simulink model "VFM_voltagesag"  (R2025a)
settings: Solver=FixedStepAuto  StartTime=0.0  StopTime=t_end+t_sim_start  FixedStep=Ts  RelTol=1e-3
InitFcn:
  | run VFMPara.m
values from neighbouring files (symbols this model uses):
  Cf = 0.0083    [GFMPara.m]    (also in GFMPara_exp.m = 0.0249; VFMPara.m = 0.02; VFMPara_exp.m = 0.03)
  dt_sag = t_c    [GFMPara.m]    (also in GFMPara_exp.m; PLLpara.m; VFMPara.m; VFMPara_exp.m)
  Lc = 1e-9    (= 1e-09)    [GFMPara.m]    (also in GFMPara_exp.m; PLLpara.m; VFMPara.m; VFMPara_exp.m)
  Lf = 0.0592    [GFMPara.m]    (also in GFMPara_exp.m; PLLpara.m = 0.05; VFMPara.m = 0.05; VFMPara_exp.m = 0.05)
  Lg11 = Xg    [PLLpara.m]    (also in VFMPara.m; VFMPara_exp.m)
  m_gfm = 1/D    [GFMPara.m]    (also in GFMPara_exp.m)
  Rg11 = Rg    [PLLpara.m]    (also in VFMPara.m; VFMPara_exp.m)
  Sbase = 1    [GFMPara.m]    (also in GFMPara_exp.m; PLLpara.m; VFMPara.m; VFMPara_exp.m)
  Scale_ki_v = 20    [GFMPara.m]    (also in GFMPara_exp.m; VFMPara.m; VFMPara_exp.m)
  t0_sag = t_sim_start +t_start    [GFMPara.m]    (also in GFMPara_exp.m; PLLpara.m = 20; VFMPara.m; VFMPara_exp.m = 20)
  Ts = 1/Fs    (= 1e-05)    [GFMPara.m]    (also in GFMPara_exp.m = 1e-06; PLLpara.m = 1e-06; VFMPara.m = 5e-06; VFMPara_exp.m = 1e-06)
  v_sag = Ug_fault    [GFMPara.m]    (also in GFMPara_exp.m; PLLpara.m; VFMPara.m; VFMPara_exp.m)
  Vbase = 1    [GFMPara.m]    (also in GFMPara_exp.m; PLLpara.m; VFMPara.m; VFMPara_exp.m)
  Vdc_ref = 2.5    [GFMPara_exp.m]
  w_droop = D/J    [GFMPara.m]    (also in GFMPara_exp.m; VFMPara.m = 314.159265359; VFMPara_exp.m = 314.159265359)
  w_i_GFM = 2000*2*pi    (= 12566.3706144)    [GFMPara.m]    (also in GFMPara_exp.m = 9424.77796077; VFMPara.m = 9424.77796077; VFMPara_exp.m = 9424.77796077)
  w_v_GFM = 800 *2*pi    (= 5026.54824574)    [GFMPara.m]    (also in GFMPara_exp.m = 3141.59265359; VFMPara.m = 3141.59265359; VFMPara_exp.m = 3141.59265359)
  Wbase = 2*pi*50    (= 314.159265359)    [GFMPara.m]    (also in GFMPara_exp.m; PLLpara.m; VFMPara.m; VFMPara_exp.m)
  Zbase = Vbase/Ibase    (= 1)    [GFMPara.m]    (also in GFMPara_exp.m; PLLpara.m; VFMPara.m; VFMPara_exp.m)
undefined symbols (not defined in the file or in its folder): DiscIntNeverNeededParam, dspblkCoreblockFVToolHelper, gcbh, initial, Kip, Kpp, Pin, Y_dc
libraries: spsVoltageMeasurementLib x32, spsCurrentMeasurementLib x30, spsControlledVoltageSourceLib x12, spsThreePhaseSeriesRLCBranchLib x9, spsSeriesRLCBranchLib x8, spsControlledCurrentSourceLib x4, spsDCVoltageSourceLib x2, spsDiodeLib x2, spspowerguiLib x1
(part 1 of 2)
settings Model: Creator=admin_user  LastModifiedBy=yifan
settings SolverCC: AlgebraicLoopSolver=TrustRegion
settings DataIOCC: ReturnWorkspaceOutputs=off
settings ModelReferenceCC: EnableRefExpFcnMdlSchedulingChecks=on
settings RTWCC: GPUComputeCapability=3.5  DLArmComputeVersion=19.05

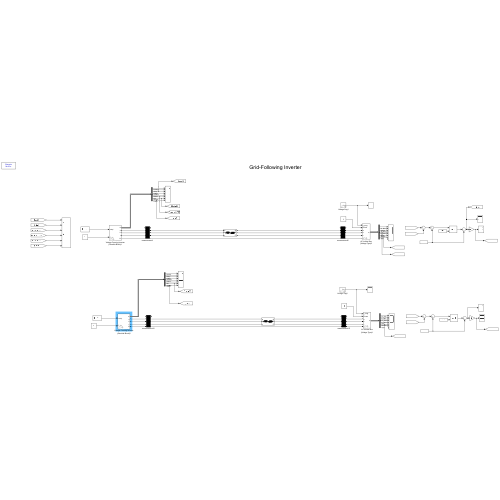
[thumbnail: Simulink's stored preview of the top-level diagram]
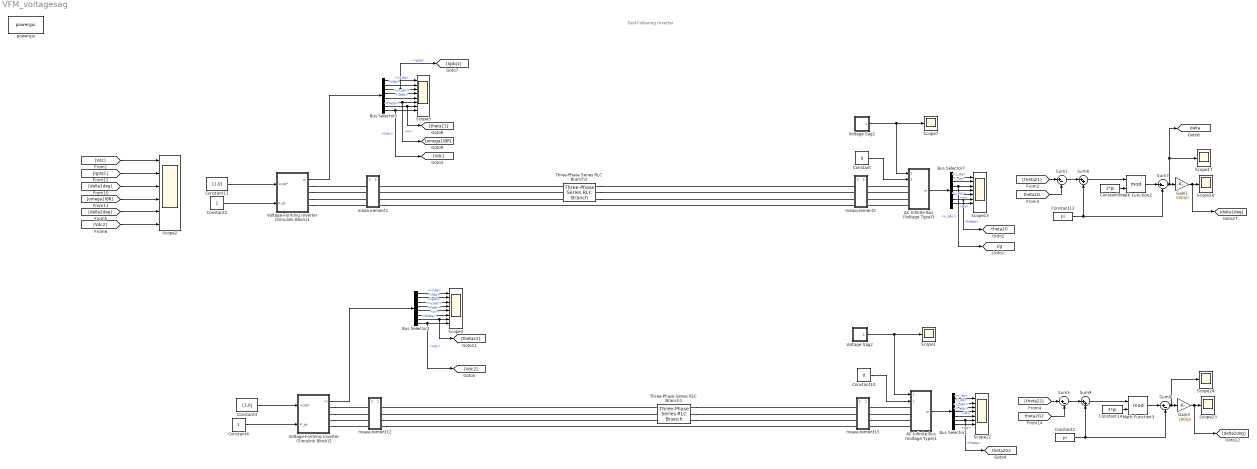
== system VFM_voltagesag ==
  note: Grid-Following Inverter
  AC Infinite Bus (Voltage Type)1 : Subsystem  AncestorBlock=|  mask{Ts=Ts, Sbase=Sbase, Vbase=Vbase, Wbase=Wbase, theta0=0, w=Wbase, R=1e-30}
      | SimplusGT/AC Infinite Bus
      | (Voltage Type)
      mask prompts: Ts "Ts (s), samping period"; Sbase "Sbase (VA), power base"; Vbase "Vbase (V), voltage base"; Wbase "Wbase (rad/s), frequency base"; theta0 "theta0 (rad), initial angle"; w "w (rad/s), frequency"; R "R (Ohm), resistance"
  AC Infinite Bus (Voltage Type)3 : Subsystem  AncestorBlock=|  mask{Ts=Ts, Sbase=Sbase, Vbase=Vbase, Wbase=Wbase, theta0=0, w=Wbase, R=1e-30}
      | SimplusGT/AC Infinite Bus
      | (Voltage Type)
      mask prompts: Ts "Ts (s), samping period"; Sbase "Sbase (VA), power base"; Vbase "Vbase (V), voltage base"; Wbase "Wbase (rad/s), frequency base"; theta0 "theta0 (rad), initial angle"; w "w (rad/s), frequency"; R "R (Ohm), resistance"
  Bus Selector1 : BusSelector  OutputSignals=v_dq,i_dq,v_abc,i_abc,w,theta,pq
  Bus Selector2 : BusSelector  OutputSignals=vcdq,ildq,igdq,vcabc,ilabc,w,theta,Vdc
  Bus Selector5 : BusSelector  OutputSignals=vcdq,ildq,igdq,vcabc,ilabc,w,theta,Vdc
  Bus Selector7 : BusSelector  OutputSignals=v_dq,i_dq,v_abc,i_abc,w,theta,pq
  Constant : Constant  Value=0
  Constant1 : Constant  Value=pi
  Constant10 : Constant  Value=0
  Constant11 : Constant  Value=[1,0]
  Constant12 : Constant  Value=pi
  Constant14 : Constant  Value=2*pi
  Constant2 : Constant
  Constant3 : Constant  Value=[1,0]
  Constant4 : Constant
  Constant9 : Constant  Value=2*pi
  Gain1 : Gain  Gain=180/pi
  Gain3 : Gain  Gain=180/pi
  Math Function2 : Math  Operator=mod  SignedPower=on
  Math Function3 : Math  Operator=mod  SignedPower=on
  Scope{1,7,16..17,23..24} (6 alike) : Scope
      Scope1 settings: ActiveDisplayYMinimum=0.9  ActiveDisplayYMaximum=1.1  DataLoggingVariableName=ScopeData15
      Scope16 settings: ActiveDisplayYMinimum=-0.045003  ActiveDisplayYMaximum=-0.044992  DataLoggingDecimation=10  DataLoggingVariableName=ScopeData6
      Scope17 settings: ActiveDisplayYMinimum=-0.00078544  ActiveDisplayYMaximum=-0.00078526  DataLoggingDecimation=10  DataLoggingVariableName=log_Delta
      Scope23 settings: ActiveDisplayYMinimum=-224.72735  ActiveDisplayYMaximum=224.86411  DataLoggingDecimation=10  DataLoggingVariableName=ScopeData7
      Scope24 settings: ActiveDisplayYMinimum=-3.92678  ActiveDisplayYMaximum=3.92693  DataLoggingDecimation=10  DataLoggingVariableName=log_Delta2
      Scope7 settings: ActiveDisplayYMinimum=0.9  ActiveDisplayYMaximum=1.1
  Scope{3,5,15,22} (4 alike) : Scope  NumInputPorts=8
      Scope15 settings: ActiveDisplayYMinimum=-0.125  ActiveDisplayYMaximum=1.125  DataLoggingVariableName=ScopeData5
      Scope22 settings: ActiveDisplayYMinimum=-0.12499999999999997  ActiveDisplayYMaximum=1.125  DataLoggingVariableName=ScopeData20
      Scope3 settings: ActiveDisplayYMinimum=-0.32470948731946192  ActiveDisplayYMaximum=1.552053078523207  DataLoggingDecimation=10  DataLoggingVariableName=ScopeData3
      Scope5 settings: ActiveDisplayYMinimum=-0.12696977606598872  ActiveDisplayYMaximum=1.1252178168649181  DataLoggingDecimation=10  DataLoggingVariableName=ScopeData2
  Scope2 : Scope  NumInputPorts=6
      settings: TimeSpan=1.5  ActiveDisplayYMinimum=1.8779617654019547  ActiveDisplayYMaximum=3.0300434734077735  DataLoggingDecimation=10
  Sum{1,5,7,9} (4 alike) : Sum  Inputs=|+-
  Sum6 : Sum  Inputs=|++
  Sum8 : Sum  Inputs=|++
  Three-Phase Series RLC Branch1 : spsThreePhaseSeriesRLCBranchLib/Three-Phase Series RLC Branch  LConnTagsString=A|B|C  RConnTagsString=A|B|C  BranchType=RL  Resistance=Rg11*Zbase  Inductance=Lg11*Zbase/Wbase  Capacitance=1/Wbase  Measurements=None
  Three-Phase Series RLC Branch2 : spsThreePhaseSeriesRLCBranchLib/Three-Phase Series RLC Branch  LConnTagsString=A|B|C  RConnTagsString=A|B|C  BranchType=RL  Resistance=Rg11*Zbase  Inductance=Lg11*Zbase/Wbase  Capacitance=1/Wbase  Measurements=None
  Voltage Sag1 : Subsystem  AncestorBlock=SimplusGT/Single Pulse  mask{t0=t0_sag, dt=dt_sag, Am=v_sag}
      mask prompts: t0 "t0 (s), starting time"; dt "dt (s), pulse width"; Am "Am, pulse amplitude"
  Voltage Sag2 : Subsystem  AncestorBlock=SimplusGT/Single Pulse  mask{t0=t0_sag, dt=dt_sag, Am=v_sag}
      mask prompts: t0 "t0 (s), starting time"; dt "dt (s), pulse width"; Am "Am, pulse amplitude"
  Voltage-Forming Inverter (Simulink Block)1 : Subsystem  AncestorBlock=|  mask{Ts=Ts, Sbase=Sbase, Vbase=Vbase, Wbase=Wbase, w_i=w_i_GFM, w_v=w_v_GFM, w_droop=w_droop*1, m=m_gfm, Lf=Lf, Cf=Cf, Lc=Lc, Scale_ki_v=Scale_ki_v}
      | SimplexPS/Grid-Forming Inverter
      | (Simulink Block)
      mask prompts: Ts "Ts (s), sampling period"; Sbase "Sbase (VA), base power"; Vbase "Vbase (V), base voltage"; Wbase "Wbase (rad/s), base frequency"; w_i "w_i (rad/s), current-loop bandwidth"; w_v "w_v (rad/s), voltage-loop bandwidth"; w_droop "w_droop (rad/s), droop bandwidth"; m "m (pu), frequency droop gain"; Lf "Lf (pu), LCL filter"; Cf "Cf (pu), LCL filter"; Lc "Lc (pu), LCL filter"
  Voltage-Forming Inverter (Simulink Block)2 : Subsystem  AncestorBlock=|  mask{Ts=Ts, Sbase=Sbase, Vbase=Vbase, Wbase=Wbase, w_i=w_i_GFM, w_v=w_v_GFM, w_droop=w_droop*1, m=m_gfm, Lf=Lf, Cf=Cf, Lc=Lc, Scale_ki_v=Scale_ki_v}
      | SimplexPS/Grid-Forming Inverter
      | (Simulink Block)
      mask prompts: Ts "Ts (s), sampling period"; Sbase "Sbase (VA), base power"; Vbase "Vbase (V), base voltage"; Wbase "Wbase (rad/s), base frequency"; w_i "w_i (rad/s), current-loop bandwidth"; w_v "w_v (rad/s), voltage-loop bandwidth"; w_droop "w_droop (rad/s), droop bandwidth"; m "m (pu), frequency droop gain"; Lf "Lf (pu), LCL filter"; Cf "Cf (pu), LCL filter"; Lc "Lc (pu), LCL filter"
  measurement1 : Subsystem
      settings: PortSchema="{\"entries\":[{\"content\":{\"sides\":[{\"content\":{\"connectorIds\":[\"Out2\",\"LConn1\",\"LConn2\",\"LConn3\",\"LConn4\"]},\"type\":\"ConnectorPlacement.EquallySpacedRectSide\",\"uuid\":\"b97639c7-89ad-4c11-8fcc-ddc4f61f4533\"},{\"content\":{\"connectorIds\":[\"Out1\",\"RConn1\",\"RConn2\",\"RConn3\",\"RConn4\"],\"side\":\"RIGHT\"},\"type\":\"ConnectorPlacement.EquallySpacedRectSide\",\"uuid\":\"3b8f0759-83d7-4d3a-a5c5-bdf29e7cbe5b\"},{\"content\":{\"connectorIds\":[],\"side\":\"TOP\"},\"type\":\"ConnectorPlacement.EquallySpacedRectSide\",\"uuid\":\"1e391932-f1e1-4127-bfe0-28b7de5de667\"},{\"content\":{\"connectorIds\":[],\"side\":\"BOTTOM\"},\"type\":\"ConnectorPlacement.EquallySpacedRectSide\",\"uuid\":\"f0c236e9-048a-4270-a45f-ff2fecf0ec8b\"}]},\"type\":\"ConnectorPlacement.EquallySpacedConnector\",\"uuid\":\"002609f8-6c16-431f-ae58-b6d94c927972\"}],\"packageUris\":[\"http://schema.mathworks.com/mf0/Connector/R2020b\"],\"version\":\"1.0\"}"
  measurement12 : Subsystem
      settings: PortSchema="{\"entries\":[{\"content\":{\"sides\":[{\"content\":{\"connectorIds\":[\"Out2\",\"LConn1\",\"LConn2\",\"LConn3\",\"LConn4\"]},\"type\":\"ConnectorPlacement.EquallySpacedRectSide\",\"uuid\":\"b97639c7-89ad-4c11-8fcc-ddc4f61f4533\"},{\"content\":{\"connectorIds\":[\"Out1\",\"RConn1\",\"RConn2\",\"RConn3\",\"RConn4\"],\"side\":\"RIGHT\"},\"type\":\"ConnectorPlacement.EquallySpacedRectSide\",\"uuid\":\"3b8f0759-83d7-4d3a-a5c5-bdf29e7cbe5b\"},{\"content\":{\"connectorIds\":[],\"side\":\"TOP\"},\"type\":\"ConnectorPlacement.EquallySpacedRectSide\",\"uuid\":\"1e391932-f1e1-4127-bfe0-28b7de5de667\"},{\"content\":{\"connectorIds\":[],\"side\":\"BOTTOM\"},\"type\":\"ConnectorPlacement.EquallySpacedRectSide\",\"uuid\":\"f0c236e9-048a-4270-a45f-ff2fecf0ec8b\"}]},\"type\":\"ConnectorPlacement.EquallySpacedConnector\",\"uuid\":\"002609f8-6c16-431f-ae58-b6d94c927972\"}],\"packageUris\":[\"http://schema.mathworks.com/mf0/Connector/R2020b\"],\"version\":\"1.0\"}"
  measurement15 : Subsystem
      settings: PortSchema="{\"entries\":[{\"content\":{\"sides\":[{\"content\":{\"connectorIds\":[\"Out2\",\"LConn1\",\"LConn2\",\"LConn3\",\"LConn4\"]},\"type\":\"ConnectorPlacement.EquallySpacedRectSide\",\"uuid\":\"b97639c7-89ad-4c11-8fcc-ddc4f61f4533\"},{\"content\":{\"connectorIds\":[\"Out1\",\"RConn1\",\"RConn2\",\"RConn3\",\"RConn4\"],\"side\":\"RIGHT\"},\"type\":\"ConnectorPlacement.EquallySpacedRectSide\",\"uuid\":\"3b8f0759-83d7-4d3a-a5c5-bdf29e7cbe5b\"},{\"content\":{\"connectorIds\":[],\"side\":\"TOP\"},\"type\":\"ConnectorPlacement.EquallySpacedRectSide\",\"uuid\":\"1e391932-f1e1-4127-bfe0-28b7de5de667\"},{\"content\":{\"connectorIds\":[],\"side\":\"BOTTOM\"},\"type\":\"ConnectorPlacement.EquallySpacedRectSide\",\"uuid\":\"f0c236e9-048a-4270-a45f-ff2fecf0ec8b\"}]},\"type\":\"ConnectorPlacement.EquallySpacedConnector\",\"uuid\":\"002609f8-6c16-431f-ae58-b6d94c927972\"}],\"packageUris\":[\"http://schema.mathworks.com/mf0/Connector/R2020b\"],\"version\":\"1.0\"}"
  measurement5 : Subsystem
      settings: PortSchema="{\"entries\":[{\"content\":{\"sides\":[{\"content\":{\"connectorIds\":[\"Out2\",\"LConn1\",\"LConn2\",\"LConn3\",\"LConn4\"]},\"type\":\"ConnectorPlacement.EquallySpacedRectSide\",\"uuid\":\"b97639c7-89ad-4c11-8fcc-ddc4f61f4533\"},{\"content\":{\"connectorIds\":[\"Out1\",\"RConn1\",\"RConn2\",\"RConn3\",\"RConn4\"],\"side\":\"RIGHT\"},\"type\":\"ConnectorPlacement.EquallySpacedRectSide\",\"uuid\":\"3b8f0759-83d7-4d3a-a5c5-bdf29e7cbe5b\"},{\"content\":{\"connectorIds\":[],\"side\":\"TOP\"},\"type\":\"ConnectorPlacement.EquallySpacedRectSide\",\"uuid\":\"1e391932-f1e1-4127-bfe0-28b7de5de667\"},{\"content\":{\"connectorIds\":[],\"side\":\"BOTTOM\"},\"type\":\"ConnectorPlacement.EquallySpacedRectSide\",\"uuid\":\"f0c236e9-048a-4270-a45f-ff2fecf0ec8b\"}]},\"type\":\"ConnectorPlacement.EquallySpacedConnector\",\"uuid\":\"002609f8-6c16-431f-ae58-b6d94c927972\"}],\"packageUris\":[\"http://schema.mathworks.com/mf0/Connector/R2020b\"],\"version\":\"1.0\"}"
  powergui : spspowerguiLib/powergui  Priority=1  SimulationMode=Discrete  SampleTime=Ts  frequency=60  Iterations=50  frequencyindice=0  Pbase=100e6  ErrMax=1e-4  UnitsV=kV  UnitsW=MW  buscounter=0  FunctionMessages=off  echomessages=off  EnableUseOfTLC=off  CurrentSourceSwitches=off  DisableSnubberDevices=off  DisableRonSwitches=off  DisableVfSwitches=off  DisplayEquations=off  AutomaticDiscreteSolvers=off  SolverType=Tustin/Backward Euler (TBE)  Interpol=off  ExternalGateDelay=off  methode=off  Ts=100  x0status=blocks  SPID=on  SwTol=0  HookPort=off  NonlinearTolerance=1e-4  nMaxIteration=100  ContinueOnMaxIteration=off  RestoreLinks=warning  ResistiveCurrentMeasurement=off  Frange=[0:2:500]  Ylog=off  Xlog=on  ShowGrid=off  save=off  variable=ZData  structure=0  ZoomFFT=off  StartTime=0.0  cycles=1  DisplayStyle=1  fundamental=60  FreqAxis=off  MaxFrequency=1000  frequencyindicesteady=1  RmsSteady=1  display=off
  tag scope: Ug=global, delta=global, theta2G2=global, theta2G=global
  wires:
  [theta21] -> Sum1/1
  Constant12/1 -> Sum6/2, Sum7/2
  Sum1/1 -> Sum6/1
  Bus Selector7/3 -> [Ug], Scope15/3  "<v_abc>"
  AC Infinite Bus (Voltage Type)3/1(m) -> Bus Selector7/1
  Constant9/1 -> Math Function2/2
  [theta2G] -> Sum1/2
  Gain1/1 -> [delta1deg], Scope16/1
  Bus Selector7/4 -> Scope15/4  "<i_abc>"
  Bus Selector7/5 -> Scope15/5  "<w>"
  Sum7/1 -> [delta], Scope17/1, Gain1/1
  Sum6/1 -> Math Function2/1
  Math Function2/1 -> Sum7/1
  Bus Selector7/7 -> Scope15/7  "<pq>"
  Bus Selector7/6 -> [theta2G], Scope15/6  "<theta>"
  Bus Selector7/1 -> Scope15/1  "<v_dq>"
  Constant/1 -> AC Infinite Bus (Voltage Type)3/2(Phase)
  Bus Selector7/2 -> Scope15/2  "<i_dq>"
  Voltage Sag1/1(Out) -> AC Infinite Bus (Voltage Type)3/1(v_mag), Scope7/1
  [delta1deg] -> Scope2/3
  Voltage-Forming Inverter (Simulink Block)1/1(m) -> Bus Selector5/1
  Bus Selector5/5 -> Scope5/5  "<ilabc>"
  Bus Selector5/4 -> Scope5/4  "<vcabc>"
  Constant11/1 -> Voltage-Forming Inverter (Simulink Block)1/1(vcdq*)
  [omega1IBR] -> Scope2/4
  Bus Selector5/1 -> Scope5/1  "<vcdq>"
  Bus Selector5/2 -> Scope5/2  "<ildq>"
  Bus Selector5/3 -> [Igdq1], Scope5/3  "<igdq>"
  [Igdq1] -> Scope2/2
  Constant2/1 -> Voltage-Forming Inverter (Simulink Block)1/2(P_dc)
  Bus Selector5/6 -> [omega1IBR], Scope5/6  "<w>"
  Bus Selector5/7 -> [theta21], Scope5/7  "<theta>"
  Bus Selector5/8 -> [Vdc], Scope5/8  "<Vdc>"
  [Vdc] -> Scope2/1
  [theta22] -> Sum5/1
  Sum5/1 -> Sum8/1
  Constant14/1 -> Math Function3/2
  Constant10/1 -> AC Infinite Bus (Voltage Type)1/2(Phase)
  Bus Selector1/4 -> Scope22/4  "<i_abc>"
  Gain3/1 -> [delta2deg], Scope23/1
  Bus Selector1/3 -> Scope22/3  "<v_abc>"
  Bus Selector1/1 -> Scope22/1  "<v_dq>"
  AC Infinite Bus (Voltage Type)1/1(m) -> Bus Selector1/1
  Math Function3/1 -> Sum9/1
  [theta2G2] -> Sum5/2
  Bus Selector1/5 -> Scope22/5  "<w>"
  Sum9/1 -> Scope24/1, Gain3/1
  Bus Selector1/7 -> Scope22/7  "<pq>"
  Constant1/1 -> Sum8/2, Sum9/2
  Sum8/1 -> Math Function3/1
  Bus Selector1/6 -> [theta2G2], Scope22/6  "<theta>"
  Bus Selector1/2 -> Scope22/2  "<i_dq>"
  Voltage Sag2/1(Out) -> AC Infinite Bus (Voltage Type)1/1(v_mag), Scope1/1
  Constant4/1 -> Voltage-Forming Inverter (Simulink Block)2/2(P_dc)
  Constant3/1 -> Voltage-Forming Inverter (Simulink Block)2/1(vcdq*)
  Bus Selector2/4 -> Scope3/4  "<vcabc>"
  Bus Selector2/8 -> [Vdc2], Scope3/8  "<Vdc>"
  Bus Selector2/7 -> [theta22], Scope3/7  "<theta>"
  Bus Selector2/2 -> Scope3/2  "<ildq>"
  Bus Selector2/1 -> Scope3/1  "<vcdq>"
  Bus Selector2/6 -> Scope3/6  "<w>"
  Bus Selector2/3 -> Scope3/3  "<igdq>"
  Bus Selector2/5 -> Scope3/5  "<ilabc>"
  Voltage-Forming Inverter (Simulink Block)2/1(m) -> Bus Selector2/1
  [delta2deg] -> Scope2/5
  [Vdc2] -> Scope2/6
  connections:
  measurement1/RConn4 -- measurement5/LConn4
  AC Infinite Bus (Voltage Type)3/LConn4 -- measurement5/RConn4
  AC Infinite Bus (Voltage Type)3/LConn1 -- measurement5/RConn1
  AC Infinite Bus (Voltage Type)3/LConn2 -- measurement5/RConn2
  AC Infinite Bus (Voltage Type)3/LConn3 -- measurement5/RConn3
  Three-Phase Series RLC Branch2/LConn1 -- measurement5/LConn1
  Three-Phase Series RLC Branch2/LConn2 -- measurement5/LConn2
  Three-Phase Series RLC Branch2/LConn3 -- measurement5/LConn3
  Three-Phase Series RLC Branch2/RConn3 -- measurement1/RConn3
  Three-Phase Series RLC Branch2/RConn2 -- measurement1/RConn2
  Three-Phase Series RLC Branch2/RConn1 -- measurement1/RConn1
  Voltage-Forming Inverter (Simulink Block)1/RConn1 -- measurement1/LConn1
  Voltage-Forming Inverter (Simulink Block)1/RConn2 -- measurement1/LConn2
  Voltage-Forming Inverter (Simulink Block)1/RConn3 -- measurement1/LConn3
  Voltage-Forming Inverter (Simulink Block)1/RConn4 -- measurement1/LConn4
  Three-Phase Series RLC Branch1/LConn2 -- measurement15/LConn2
  Three-Phase Series RLC Branch1/LConn1 -- measurement15/LConn1
  Three-Phase Series RLC Branch1/LConn3 -- measurement15/LConn3
  measurement12/RConn4 -- measurement15/LConn4
  AC Infinite Bus (Voltage Type)1/LConn1 -- measurement15/RConn1
  AC Infinite Bus (Voltage Type)1/LConn2 -- measurement15/RConn2
  AC Infinite Bus (Voltage Type)1/LConn3 -- measurement15/RConn3
  Three-Phase Series RLC Branch1/RConn1 -- measurement12/RConn1
  Three-Phase Series RLC Branch1/RConn3 -- measurement12/RConn3
  AC Infinite Bus (Voltage Type)1/LConn4 -- measurement15/RConn4
  Three-Phase Series RLC Branch1/RConn2 -- measurement12/RConn2
  Voltage-Forming Inverter (Simulink Block)2/RConn1 -- measurement12/LConn1
  Voltage-Forming Inverter (Simulink Block)2/RConn3 -- measurement12/LConn3
  Voltage-Forming Inverter (Simulink Block)2/RConn4 -- measurement12/LConn4
  Voltage-Forming Inverter (Simulink Block)2/RConn2 -- measurement12/LConn2

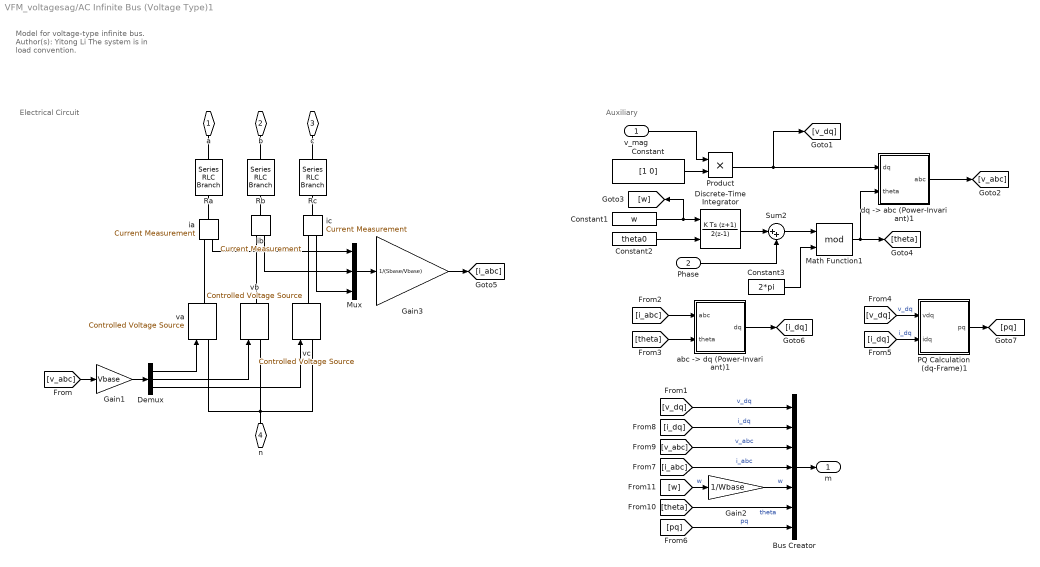
== system VFM_voltagesag/AC Infinite Bus (Voltage Type)1 ==
  note: Auxiliary
  note: Electrical Circuit
  note: Model for voltage-type infinite bus.
      |
      | Author(s): Yitong Li
      |
      | The system is in load convention.
  v_mag : Inport
  Phase : Inport  Port=2
  Bus Creator : BusCreator  Inputs=7
  Constant : Constant  Value=[1 0]
  Constant1 : Constant  Value=w
  Constant2 : Constant  Value=theta0
  Constant3 : Constant  Value=2*pi
  Demux : Demux  Outputs=3
  Discrete-Time Integrator : DiscreteIntegrator  IntegratorMethod=Integration: Trapezoidal  InitialConditionSource=external  SampleTime=-1  ICPrevOutput=DiscIntNeverNeededParam  ICPrevScaledInput=DiscIntNeverNeededParam
  Gain1 : Gain  Gain=Vbase
  Gain2 : Gain  Gain=1/Wbase
  Gain3 : Gain  Gain=1/(Sbase/Vbase)
  Math Function1 : Math  Operator=mod  SignedPower=on
  Mux : Mux  Inputs=3
  PQ Calculation (dq-Frame)1 : Subsystem  AncestorBlock=|
      | SimplusGT/PQ Calculation
      | (dq-Frame)
  Product : Product
  Ra : spsSeriesRLCBranchLib/Series RLC Branch  LConnTagsString=__new0  RConnTagsString=__new0  BranchType=R  Resistance=R  Inductance=1e-3  SetiL0=off  InitialCurrent=0  Capacitance=1e-6  Setx0=off  InitialVoltage=0  Measurements=None
  Rb : spsSeriesRLCBranchLib/Series RLC Branch  LConnTagsString=__new0  RConnTagsString=__new0  BranchType=R  Resistance=R  Inductance=1e-3  SetiL0=off  InitialCurrent=0  Capacitance=1e-6  Setx0=off  InitialVoltage=0  Measurements=None
  Rc : spsSeriesRLCBranchLib/Series RLC Branch  LConnTagsString=__new0  RConnTagsString=__new0  BranchType=R  Resistance=R  Inductance=1e-3  SetiL0=off  InitialCurrent=0  Capacitance=1e-6  Setx0=off  InitialVoltage=0  Measurements=None
  Sum2 : Sum  Inputs=|++
  "abc -> dq (Power-Invariant)1" : Subsystem  AncestorBlock=|
      | SimplusGT/abc -> dq
      | (Power-Invariant)
  "dq -> abc (Power-Invariant)1" : Subsystem  AncestorBlock=|
      | SimplusGT/dq -> abc
      | (Power-Invariant)
  ia : spsCurrentMeasurementLib/Current Measurement  PhasorSimulation=off  OutputType=Complex  PSBequivalent=0
  ib : spsCurrentMeasurementLib/Current Measurement  PhasorSimulation=off  OutputType=Complex  PSBequivalent=0
  ic : spsCurrentMeasurementLib/Current Measurement  PhasorSimulation=off  OutputType=Complex  PSBequivalent=0
  va : spsControlledVoltageSourceLib/Controlled Voltage Source  Initialize=on  Source_Type=AC  Amplitude=0  Phase=0  Frequency=0  Measurements=None
  vb : spsControlledVoltageSourceLib/Controlled Voltage Source  Initialize=on  Source_Type=AC  Amplitude=0  Phase=0  Frequency=0  Measurements=None
  vc : spsControlledVoltageSourceLib/Controlled Voltage Source  Initialize=on  Source_Type=AC  Amplitude=0  Phase=0  Frequency=0  Measurements=None
  a : PMIOPort  Side=Left
  b : PMIOPort  Port=2  Side=Left
  c : PMIOPort  Port=3  Side=Left
  n : PMIOPort  Port=4  Side=Left
  m : Outport
  wires:
  [pq] -> Bus Creator/7  "pq"
  PQ Calculation (dq-Frame)1/1(pq) -> [pq]
  [i_dq] -> PQ Calculation (dq-Frame)1/2(idq)  "i_dq"
  [v_dq] -> PQ Calculation (dq-Frame)1/1(vdq)  "v_dq"
  Gain3/1 -> [i_abc]
  Mux/1 -> Gain3/1
  Gain1/1 -> Demux/1
  "abc -> dq (Power-Invariant)1"/1(dq) -> [i_dq]
  [theta] -> "abc -> dq (Power-Invariant)1"/2(theta)
  [i_abc] -> "abc -> dq (Power-Invariant)1"/1(abc)
  ic/1 -> Mux/3
  ib/1 -> Mux/2
  ia/1 -> Mux/1
  [theta] -> Bus Creator/6  "theta"
  Bus Creator/1 -> m/1
  [i_dq] -> Bus Creator/2  "i_dq"
  Gain2/1 -> Bus Creator/5  "w"
  [v_abc] -> Bus Creator/3  "v_abc"
  [w] -> Gain2/1  "w"
  [i_abc] -> Bus Creator/4  "i_abc"
  [v_dq] -> Bus Creator/1  "v_dq"
  Constant3/1 -> Math Function1/2
  "dq -> abc (Power-Invariant)1"/1(abc) -> [v_abc]
  Constant1/1 -> [w], Discrete-Time Integrator/1
  Constant2/1 -> Discrete-Time Integrator/2
  Math Function1/1 -> [theta], "dq -> abc (Power-Invariant)1"/2(theta)
  Demux/3 -> vc/1
  Demux/2 -> vb/1
  Demux/1 -> va/1
  [v_abc] -> Gain1/1
  Constant/1 -> Product/2
  v_mag/1 -> Product/1
  Product/1 -> [v_dq], "dq -> abc (Power-Invariant)1"/1(dq)
  Discrete-Time Integrator/1 -> Sum2/1
  Sum2/1 -> Math Function1/1
  Phase/1 -> Sum2/2
  connections:
  Rc/LConn1 -- c/RConn1
  Rc/RConn1 -- ic/LConn1
  Rb/LConn1 -- b/RConn1
  ib/LConn1 -- Rb/RConn1
  Ra/LConn1 -- a/RConn1
  Ra/RConn1 -- ia/LConn1
  ic/RConn1 -- vc/RConn1
  ib/RConn1 -- vb/RConn1
  ia/RConn1 -- va/RConn1
  vb/LConn1 -- va/LConn1 -- n/RConn1 -- vc/LConn1

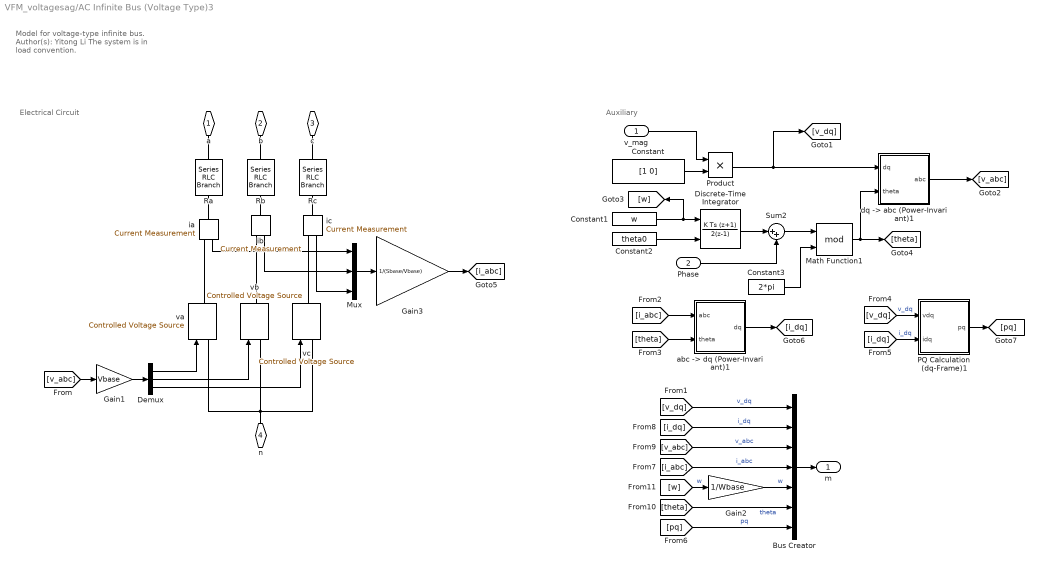
== system VFM_voltagesag/AC Infinite Bus (Voltage Type)3 ==
  note: Auxiliary
  note: Electrical Circuit
  note: Model for voltage-type infinite bus.
      |
      | Author(s): Yitong Li
      |
      | The system is in load convention.
  v_mag : Inport
  Phase : Inport  Port=2
  Bus Creator : BusCreator  Inputs=7
  Constant : Constant  Value=[1 0]
  Constant1 : Constant  Value=w
  Constant2 : Constant  Value=theta0
  Constant3 : Constant  Value=2*pi
  Demux : Demux  Outputs=3
  Discrete-Time Integrator : DiscreteIntegrator  IntegratorMethod=Integration: Trapezoidal  InitialConditionSource=external  SampleTime=-1  ICPrevOutput=DiscIntNeverNeededParam  ICPrevScaledInput=DiscIntNeverNeededParam
  Gain1 : Gain  Gain=Vbase
  Gain2 : Gain  Gain=1/Wbase
  Gain3 : Gain  Gain=1/(Sbase/Vbase)
  Math Function1 : Math  Operator=mod  SignedPower=on
  Mux : Mux  Inputs=3
  PQ Calculation (dq-Frame)1 : Subsystem  AncestorBlock=|
      | SimplusGT/PQ Calculation
      | (dq-Frame)
  Product : Product
  Ra : spsSeriesRLCBranchLib/Series RLC Branch  LConnTagsString=__new0  RConnTagsString=__new0  BranchType=R  Resistance=R  Inductance=1e-3  SetiL0=off  InitialCurrent=0  Capacitance=1e-6  Setx0=off  InitialVoltage=0  Measurements=None
  Rb : spsSeriesRLCBranchLib/Series RLC Branch  LConnTagsString=__new0  RConnTagsString=__new0  BranchType=R  Resistance=R  Inductance=1e-3  SetiL0=off  InitialCurrent=0  Capacitance=1e-6  Setx0=off  InitialVoltage=0  Measurements=None
  Rc : spsSeriesRLCBranchLib/Series RLC Branch  LConnTagsString=__new0  RConnTagsString=__new0  BranchType=R  Resistance=R  Inductance=1e-3  SetiL0=off  InitialCurrent=0  Capacitance=1e-6  Setx0=off  InitialVoltage=0  Measurements=None
  Sum2 : Sum  Inputs=|++
  "abc -> dq (Power-Invariant)1" : Subsystem  AncestorBlock=|
      | SimplusGT/abc -> dq
      | (Power-Invariant)
  "dq -> abc (Power-Invariant)1" : Subsystem  AncestorBlock=|
      | SimplusGT/dq -> abc
      | (Power-Invariant)
  ia : spsCurrentMeasurementLib/Current Measurement  PhasorSimulation=off  OutputType=Complex  PSBequivalent=0
  ib : spsCurrentMeasurementLib/Current Measurement  PhasorSimulation=off  OutputType=Complex  PSBequivalent=0
  ic : spsCurrentMeasurementLib/Current Measurement  PhasorSimulation=off  OutputType=Complex  PSBequivalent=0
  va : spsControlledVoltageSourceLib/Controlled Voltage Source  Initialize=on  Source_Type=AC  Amplitude=0  Phase=0  Frequency=0  Measurements=None
  vb : spsControlledVoltageSourceLib/Controlled Voltage Source  Initialize=on  Source_Type=AC  Amplitude=0  Phase=0  Frequency=0  Measurements=None
  vc : spsControlledVoltageSourceLib/Controlled Voltage Source  Initialize=on  Source_Type=AC  Amplitude=0  Phase=0  Frequency=0  Measurements=None
  a : PMIOPort  Side=Left
  b : PMIOPort  Port=2  Side=Left
  c : PMIOPort  Port=3  Side=Left
  n : PMIOPort  Port=4  Side=Left
  m : Outport
  wires:
  [pq] -> Bus Creator/7  "pq"
  PQ Calculation (dq-Frame)1/1(pq) -> [pq]
  [i_dq] -> PQ Calculation (dq-Frame)1/2(idq)  "i_dq"
  [v_dq] -> PQ Calculation (dq-Frame)1/1(vdq)  "v_dq"
  Gain3/1 -> [i_abc]
  Mux/1 -> Gain3/1
  Gain1/1 -> Demux/1
  "abc -> dq (Power-Invariant)1"/1(dq) -> [i_dq]
  [theta] -> "abc -> dq (Power-Invariant)1"/2(theta)
  [i_abc] -> "abc -> dq (Power-Invariant)1"/1(abc)
  ic/1 -> Mux/3
  ib/1 -> Mux/2
  ia/1 -> Mux/1
  [theta] -> Bus Creator/6  "theta"
  Bus Creator/1 -> m/1
  [i_dq] -> Bus Creator/2  "i_dq"
  Gain2/1 -> Bus Creator/5  "w"
  [v_abc] -> Bus Creator/3  "v_abc"
  [w] -> Gain2/1  "w"
  [i_abc] -> Bus Creator/4  "i_abc"
  [v_dq] -> Bus Creator/1  "v_dq"
  Constant3/1 -> Math Function1/2
  "dq -> abc (Power-Invariant)1"/1(abc) -> [v_abc]
  Constant1/1 -> [w], Discrete-Time Integrator/1
  Constant2/1 -> Discrete-Time Integrator/2
  Math Function1/1 -> [theta], "dq -> abc (Power-Invariant)1"/2(theta)
  Demux/3 -> vc/1
  Demux/2 -> vb/1
  Demux/1 -> va/1
  [v_abc] -> Gain1/1
  Constant/1 -> Product/2
  v_mag/1 -> Product/1
  Product/1 -> [v_dq], "dq -> abc (Power-Invariant)1"/1(dq)
  Discrete-Time Integrator/1 -> Sum2/1
  Sum2/1 -> Math Function1/1
  Phase/1 -> Sum2/2
  connections:
  Rc/LConn1 -- c/RConn1
  Rc/RConn1 -- ic/LConn1
  Rb/LConn1 -- b/RConn1
  ib/LConn1 -- Rb/RConn1
  Ra/LConn1 -- a/RConn1
  Ra/RConn1 -- ia/LConn1
  ic/RConn1 -- vc/RConn1
  ib/RConn1 -- vb/RConn1
  ia/RConn1 -- va/RConn1
  vb/LConn1 -- va/LConn1 -- n/RConn1 -- vc/LConn1

== system VFM_voltagesag/Voltage Sag1 ==
  note: Pulse generator
      |
      | Author(s): Yitong Li
  Constant : Constant
  Gain : Gain  Gain=1-Am
  Product : Product
  Step : Step  Time=t0  SampleTime=0
  Step1 : Step  Time=t0+dt  Before=1  After=0  SampleTime=0
  Subtract : Sum  Inputs=+-
  Out : Outport
  wires:
  Step1/1 -> Product/2
  Step/1 -> Product/1
  Product/1 -> Gain/1
  Gain/1 -> Subtract/2
  Subtract/1 -> Out/1
  Constant/1 -> Subtract/1

== system VFM_voltagesag/Voltage Sag2 ==
  note: Pulse generator
      |
      | Author(s): Yitong Li
  Constant : Constant
  Gain : Gain  Gain=1-Am
  Product : Product
  Step : Step  Time=t0  SampleTime=0
  Step1 : Step  Time=t0+dt  Before=1  After=0  SampleTime=0
  Subtract : Sum  Inputs=+-
  Out : Outport
  wires:
  Step1/1 -> Product/2
  Step/1 -> Product/1
  Product/1 -> Gain/1
  Gain/1 -> Subtract/2
  Subtract/1 -> Out/1
  Constant/1 -> Subtract/1

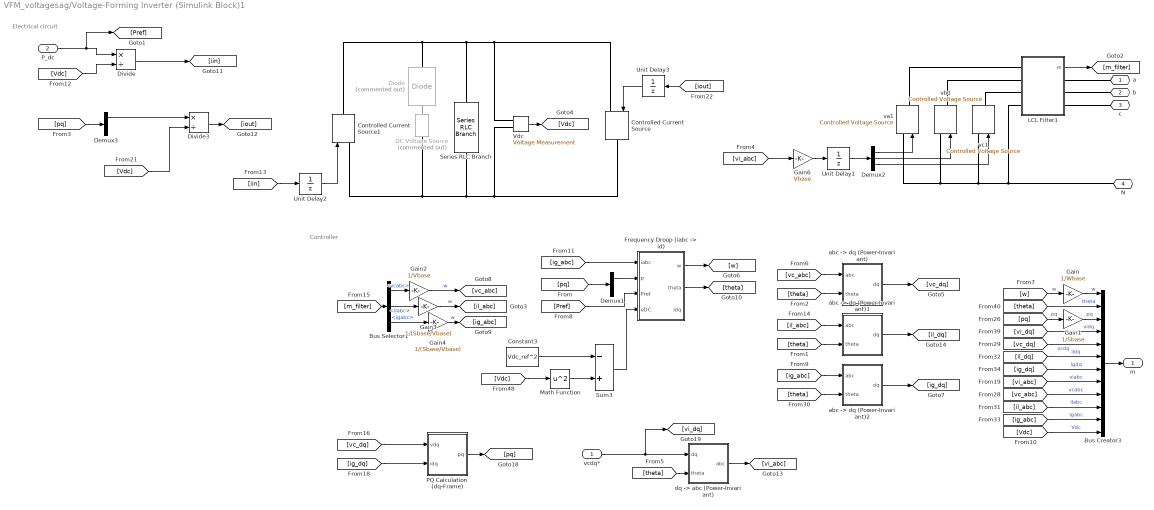
== system VFM_voltagesag/Voltage-Forming Inverter (Simulink Block)1 ==
  note: Controller
  note: Electrical circuit
  vcdq* : Inport
  P_dc : Inport  Port=2
  Bus Creator3 : BusCreator  Inputs=12
  Bus Selector1 : BusSelector  OutputSignals=vcabc,ilabc,igabc
  Constant3 : Constant  Value=Vdc_ref^2
  Controlled Current Source : spsControlledCurrentSourceLib/Controlled Current Source  Initialize=on  Source_Type=AC  Amplitude=0  Phase=0  Frequency=0  Measurements=None
  Controlled Current Source1 : spsControlledCurrentSourceLib/Controlled Current Source  Initialize=on  Source_Type=AC  Amplitude=0  Phase=0  Frequency=0  Measurements=None
  DC Voltage Source : spsDCVoltageSourceLib/DC Voltage Source  Commented=on  Amplitude=Vdc_ref  Measurements=None
  Demux1 : Demux  Outputs=2
  Demux2 : Demux  Outputs=3
  Demux3 : Demux  Outputs=2
  Diode : spsDiodeLib/Diode  Commented=on  Ron=0.01  Lon=0  Vf=0  IC=0  UseSnubber=0  Rs=1000  Cs=250e-9  Measurements=off
  Divide : Product  Inputs=*/
  Divide3 : Product  Inputs=*/
  "Frequency Droop (iabc -> id)" : Subsystem  AncestorBlock=|  mask{Ts=Ts, Sbase=Sbase, Vbase=Vbase, Wbase=Wbase, m=m, w_tau=w_droop, theta0=0, i0=Pin, w0=1}
      | SimplexPS/Frequency Droop
      | (iabc -> id)
      mask prompts: Ts "Ts (s), samping period"; Sbase "Sbase (VA), base power"; Vbase "Vbase (V), base voltage"; Wbase "Wbase (rad/s), base angular frequency"; m "m (pu), droop gain"; w_tau "w_tau (rad/s), low-pass filter bandwidth"; theta0 "theta0 (rad), initial angle"; i0 "i0 (pu), current setting point"; w0 "w0 (pu), frequency setting point"
  Gain : Gain  Gain=1/Wbase
  Gain1 : Gain  Gain=1/Sbase
  Gain2 : Gain  Gain=1/Vbase
  Gain3 : Gain  Gain=1/(Sbase/Vbase)
  Gain4 : Gain  Gain=1/(Sbase/Vbase)
  Gain6 : Gain  Gain=Vbase
  LCL Filter1 : Subsystem  mask{Lf=1e-9*(Vbase^2/Sbase)/Wbase, Rf=1e-9*(Vbase^2/Sbase), Lc=1e-9*(Vbase^2/Sbase)/Wbase, Rc=1e-9*(Vbase^2/Sbase), Cf=Cf*(Sbase/Vbase^2)/Wbase, Rd=1e-9*(Vbase^2/Sbase)}
      mask prompts: Lf "Lf (H)"; Rf "Rf (Ohm)"; Lc "Lc (H)"; Rc "Rc (Ohm)"; Cf "Cf (F)"; Rd "Rd (Ohm)"
  Math Function : Math  Operator=square
  PQ Calculation (dq-Frame) : Subsystem
  Series RLC Branch : spsSeriesRLCBranchLib/Series RLC Branch  LConnTagsString=__new0  RConnTagsString=__new0  BranchType=RC  Resistance=1e-10*(Vbase^2/Sbase)  Inductance=1e-3  SetiL0=off  InitialCurrent=0  Capacitance=Y_dc*(Sbase/Vbase^2)/Wbase  Setx0=on  InitialVoltage=Vdc_ref  Measurements=None
  Sum3 : Sum  Inputs=-+
  Unit Delay1 : UnitDelay  SampleTime=Ts  HasFrameUpgradeWarning=on
  Unit Delay2 : UnitDelay  SampleTime=-1  HasFrameUpgradeWarning=on
  Unit Delay3 : UnitDelay  SampleTime=-1  HasFrameUpgradeWarning=on
  Vdc : spsVoltageMeasurementLib/Voltage Measurement  PhasorSimulation=off  OutputType=Complex  PSBequivalent=0
  "abc -> dq (Power-Invariant)" : Subsystem
  "abc -> dq (Power-Invariant)1" : Subsystem
  "abc -> dq (Power-Invariant)2" : Subsystem
  "dq -> abc (Power-Invariant)" : Subsystem
  va1 : spsControlledVoltageSourceLib/Controlled Voltage Source  Initialize=on  Source_Type=AC  Amplitude=0  Phase=0  Frequency=0  Measurements=None
  vb1 : spsControlledVoltageSourceLib/Controlled Voltage Source  Initialize=on  Source_Type=AC  Amplitude=0  Phase=0  Frequency=0  Measurements=None
  vc1 : spsControlledVoltageSourceLib/Controlled Voltage Source  Initialize=on  Source_Type=AC  Amplitude=0  Phase=0  Frequency=0  Measurements=None
  a : PMIOPort  Side=Right
  b : PMIOPort  Port=2  Side=Right
  c : PMIOPort  Port=3  Side=Right
  N : PMIOPort  Port=4  Side=Right
  m : Outport
  wires:
  [ig_abc] -> Bus Creator3/11  "igabc"
  [il_abc] -> Bus Creator3/10  "ilabc"
  [vc_abc] -> Bus Creator3/9  "vcabc"
  [vi_abc] -> Bus Creator3/8  "viabc"
  [ig_dq] -> Bus Creator3/7  "igdq"
  [il_dq] -> Bus Creator3/6  "ildq"
  [vc_dq] -> Bus Creator3/5  "vcdq"
  [vi_dq] -> Bus Creator3/4  "vidq"
  Gain1/1 -> Bus Creator3/3  "pq"
  [theta] -> Bus Creator3/2  "theta"
  Gain/1 -> Bus Creator3/1  "w"
  [pq] -> Gain1/1  "pq"
  [w] -> Gain/1  "w"
  "abc -> dq (Power-Invariant)1"/1(dq) -> [il_dq]
  "abc -> dq (Power-Invariant)2"/1(dq) -> [ig_dq]
  "abc -> dq (Power-Invariant)"/1(dq) -> [vc_dq]
  [ig_abc] -> "Frequency Droop (iabc -> id)"/1(iabc)
  [ig_dq] -> PQ Calculation (dq-Frame)/2(idq)
  PQ Calculation (dq-Frame)/1(pq) -> [pq]
  [vc_dq] -> PQ Calculation (dq-Frame)/1(vdq)
  [theta] -> "dq -> abc (Power-Invariant)"/2(theta)
  vcdq*/1 -> "dq -> abc (Power-Invariant)"/1(dq), [vi_dq]
  "Frequency Droop (iabc -> id)"/1(w) -> [w]
  "Frequency Droop (iabc -> id)"/2(theta) -> [theta]
  [theta] -> "abc -> dq (Power-Invariant)2"/2(theta)
  [ig_abc] -> "abc -> dq (Power-Invariant)2"/1(abc)
  [il_abc] -> "abc -> dq (Power-Invariant)1"/1(abc)
  [vc_abc] -> "abc -> dq (Power-Invariant)"/1(abc)
  [theta] -> "abc -> dq (Power-Invariant)1"/2(theta)
  [theta] -> "abc -> dq (Power-Invariant)"/2(theta)
  Bus Creator3/1 -> m/1
  "dq -> abc (Power-Invariant)"/1(abc) -> [vi_abc]
  Demux1/1 -> "Frequency Droop (iabc -> id)"/2(p)
  [pq] -> Demux1/1
  Bus Selector1/3 -> Gain4/1  "<igabc>"
  Bus Selector1/2 -> Gain3/1  "<ilabc>"
  Bus Selector1/1 -> Gain2/1  "<vcabc>"
  Gain4/1 -> [ig_abc]  "w"
  [m_filter] -> Bus Selector1/1
  Gain2/1 -> [vc_abc]  "w"
  Gain3/1 -> [il_abc]  "w"
  P_dc/1 -> [Pref], Divide/1
  Vdc/1 -> [Vdc]
  [iout] -> Unit Delay3/1
  Divide3/1 -> [iout]
  [iin] -> Unit Delay2/1
  LCL Filter1/1(m) -> [m_filter]
  Divide/1 -> [iin]
  Demux2/2 -> vb1/1
  Gain6/1 -> Unit Delay1/1
  Unit Delay3/1 -> Controlled Current Source/1
  Demux2/3 -> vc1/1
  Unit Delay1/1 -> Demux2/1
  Unit Delay2/1 -> Controlled Current Source1/1
  Demux2/1 -> va1/1
  [Vdc] -> Divide3/2
  [Vdc] -> Divide/2
  [pq] -> Demux3/1
  Demux3/1 -> Divide3/1
  [Pref] -> "Frequency Droop (iabc -> id)"/3(Pref)
  Math Function/1 -> Sum3/2
  Constant3/1 -> Sum3/1
  [Vdc] -> Math Function/1
  Sum3/1 -> "Frequency Droop (iabc -> id)"/4(eDC)
  [Vdc] -> Bus Creator3/12  "Vdc"
  [vi_abc] -> Gain6/1
  connections:
  Series RLC Branch/LConn1 -- Diode/RConn1 -- Controlled Current Source1/RConn1 -- Vdc/LConn1 -- Controlled Current Source/LConn1
  va1/LConn1 -- LCL Filter1/LConn4 -- N/RConn1 -- vc1/LConn1 -- vb1/LConn1
  Series RLC Branch/RConn1 -- Controlled Current Source1/LConn1 -- DC Voltage Source/LConn1 -- Controlled Current Source/RConn1 -- Vdc/LConn2
  LCL Filter1/LConn2 -- vb1/RConn1
  LCL Filter1/RConn1 -- a/RConn1
  LCL Filter1/LConn3 -- vc1/RConn1
  LCL Filter1/LConn1 -- va1/RConn1
  LCL Filter1/RConn2 -- b/RConn1
  LCL Filter1/RConn3 -- c/RConn1
  Diode/LConn1 -- DC Voltage Source/RConn1

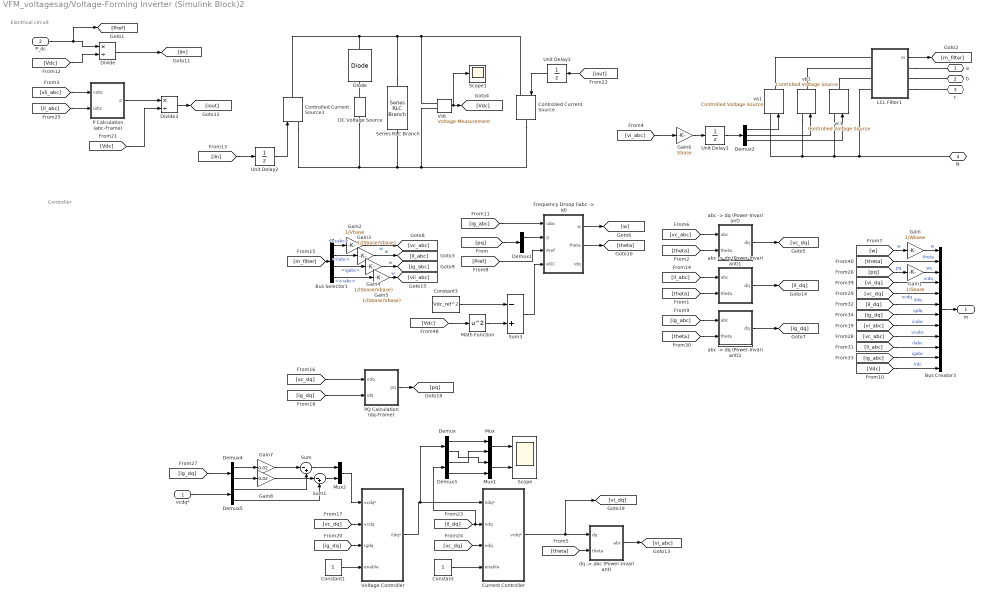
== system VFM_voltagesag/Voltage-Forming Inverter (Simulink Block)2 ==
  note: Controller
  note: Electrical circuit
  vcdq* : Inport
  P_dc : Inport  Port=2
  Bus Creator3 : BusCreator  Inputs=12
  Bus Selector1 : BusSelector  OutputSignals=vcabc,ilabc,igabc,viiabc
  Constant : Constant
  Constant1 : Constant
  Constant3 : Constant  Value=Vdc_ref^2
  Controlled Current Source : spsControlledCurrentSourceLib/Controlled Current Source  Initialize=on  Source_Type=AC  Amplitude=0  Phase=0  Frequency=0  Measurements=None
  Controlled Current Source1 : spsControlledCurrentSourceLib/Controlled Current Source  Initialize=on  Source_Type=AC  Amplitude=0  Phase=0  Frequency=0  Measurements=None
  Current Controller : Subsystem  mask{Ts=Ts, Wbase=Wbase, Lf=Lf/Wbase, Kg=0, Kp=w_i*Lf/Wbase*2, Ki=w_i*w_i/4*Lf/Wbase, xdmax=inf, xqmax=inf, Kcd=0}
      mask prompts: Ts "Sampling Time (s)"; Wbase "Base Angular Frequency (rad/s)"; Lf "Inductance"; Kg "Estimator Gain"; Kp "Proportional Gain"; Ki "Integral Gain"; xdmax "Voltage D Limit"; xqmax "Voltage Q Limit"; Kcd "Cross Decoupling Gain"
  DC Voltage Source : spsDCVoltageSourceLib/DC Voltage Source  Amplitude=3.25  Measurements=None
  Demux{,1,3..5} (5 alike) : Demux  Outputs=2
  Demux2 : Demux  Outputs=3
  Diode : spsDiodeLib/Diode  Ron=0.01  Lon=0  Vf=0  IC=0  UseSnubber=0  Rs=1e6  Cs=inf  Measurements=off
  Divide : Product  Inputs=*/
  Divide3 : Product  Inputs=*/
  "Frequency Droop (iabc -> id)" : Subsystem  AncestorBlock=|  mask{Ts=Ts, Sbase=Sbase, Vbase=Vbase, Wbase=Wbase, m=m, w_tau=w_droop, theta0=0, i0=Pin, w0=1}
      | SimplexPS/Frequency Droop
      | (iabc -> id)
      mask prompts: Ts "Ts (s), samping period"; Sbase "Sbase (VA), base power"; Vbase "Vbase (V), base voltage"; Wbase "Wbase (rad/s), base angular frequency"; m "m (pu), droop gain"; w_tau "w_tau (rad/s), low-pass filter bandwidth"; theta0 "theta0 (rad), initial angle"; i0 "i0 (pu), current setting point"; w0 "w0 (pu), frequency setting point"
  Gain : Gain  Gain=1/Wbase
  Gain1 : Gain  Gain=1/Sbase
  Gain2 : Gain  Gain=1/Vbase
  Gain3 : Gain  Gain=1/(Sbase/Vbase)
  Gain4 : Gain  Gain=1/(Sbase/Vbase)
  Gain5 : Gain  Gain=1/(Sbase/Vbase)
  Gain6 : Gain  Gain=Vbase
  Gain7 : Gain  Gain=0.02
  Gain8 : Gain  Gain=0.02
  LCL Filter1 : Subsystem  mask{Lf=Lf*(Vbase^2/Sbase)/Wbase, Rf=Lf*(Vbase^2/Sbase)*2e-6, Lc=1e-9*(Vbase^2/Sbase)/Wbase, Rc=1e-9*(Vbase^2/Sbase), Cf=Cf*(Sbase/Vbase^2)/Wbase, Rd=1e-3*(Vbase^2/Sbase)}
      mask prompts: Lf "Lf (H)"; Rf "Rf (Ohm)"; Lc "Lc (H)"; Rc "Rc (Ohm)"; Cf "Cf (F)"; Rd "Rd (Ohm)"
  Math Function : Math  Operator=square
  Mux : Mux  Inputs=2
  Mux1 : Mux  Inputs=2
  Mux2 : Mux  Inputs=2
  P Calculation (abc-Frame) : Subsystem
  PQ Calculation (dq-Frame) : Subsystem
  Scope : Scope  NumInputPorts=2
      settings: ActiveDisplayYMinimum=-0.33464461434412296  ActiveDisplayYMaximum=1.613093583112561  DataLoggingVariableName=ScopeData4
  Scope1 : Scope
      settings: ActiveDisplayYMinimum=2.0924827237669028  ActiveDisplayYMaximum=4.2567675140943511  DataLoggingVariableName=ScopeData8
  Series RLC Branch : spsSeriesRLCBranchLib/Series RLC Branch  LConnTagsString=__new0  RConnTagsString=__new0  BranchType=RC  Resistance=1e-10*(Vbase^2/Sbase)  Inductance=1e-3  SetiL0=off  InitialCurrent=0  Capacitance=Y_dc*(Sbase/Vbase^2)/Wbase  Setx0=on  InitialVoltage=Vdc_ref  Measurements=None
  Sum : Sum  Inputs=|-+
  Sum1 : Sum  Inputs=|-+
  Sum3 : Sum  Inputs=-+
  Unit Delay1 : UnitDelay  SampleTime=Ts  HasFrameUpgradeWarning=on
  Unit Delay2 : UnitDelay  SampleTime=-1  HasFrameUpgradeWarning=on
  Unit Delay3 : UnitDelay  SampleTime=-1  HasFrameUpgradeWarning=on
  Vdc : spsVoltageMeasurementLib/Voltage Measurement  PhasorSimulation=off  OutputType=Complex  PSBequivalent=0
  Voltage Controller : Subsystem  mask{Ts=Ts, Wbase=Wbase, Cf=Cf/Wbase, Kg=0, Kp=w_v*Cf/Wbase, Ki=w_v*w_v/4*Cf/Wbase*Scale_ki_v, xdmax=inf, xqmax=inf, Kcd=0}
      mask prompts: Ts "Sampling Time (s)"; Wbase "Base Angular Frequency (rad/s)"; Cf "Capacitance"; Kg "Estimator Gain"; Kp "Proportional Gain"; Ki "Integral Gain"; xdmax "Current D Limit"; xqmax "Current Q Limit"; Kcd "Cross Decoupling Gain"
  "abc -> dq (Power-Invariant)" : Subsystem
  "abc -> dq (Power-Invariant)1" : Subsystem
  "abc -> dq (Power-Invariant)2" : Subsystem
  "dq -> abc (Power-Invariant)" : Subsystem
  va1 : spsControlledVoltageSourceLib/Controlled Voltage Source  Initialize=on  Source_Type=AC  Amplitude=0  Phase=0  Frequency=0  Measurements=None
  vb1 : spsControlledVoltageSourceLib/Controlled Voltage Source  Initialize=on  Source_Type=AC  Amplitude=0  Phase=0  Frequency=0  Measurements=None
  vc1 : spsControlledVoltageSourceLib/Controlled Voltage Source  Initialize=on  Source_Type=AC  Amplitude=0  Phase=0  Frequency=0  Measurements=None
  a : PMIOPort  Side=Right
  b : PMIOPort  Port=2  Side=Right
  c : PMIOPort  Port=3  Side=Right
  N : PMIOPort  Port=4  Side=Right
  m : Outport
  wires:
  [ig_abc] -> Bus Creator3/11  "igabc"
  [il_abc] -> Bus Creator3/10  "ilabc"
  [vc_abc] -> Bus Creator3/9  "vcabc"
  [vi_abc] -> Bus Creator3/8  "viabc"
  [ig_dq] -> Bus Creator3/7  "igdq"
  [il_dq] -> Bus Creator3/6  "ildq"
  [vc_dq] -> Bus Creator3/5  "vcdq"
  [vi_dq] -> Bus Creator3/4  "vidq"
  Gain1/1 -> Bus Creator3/3  "pq"
  [theta] -> Bus Creator3/2  "theta"
  Gain/1 -> Bus Creator3/1  "w"
  [pq] -> Gain1/1  "pq"
  [w] -> Gain/1  "w"
  "abc -> dq (Power-Invariant)1"/1(dq) -> [il_dq]
  "abc -> dq (Power-Invariant)2"/1(dq) -> [ig_dq]
  "abc -> dq (Power-Invariant)"/1(dq) -> [vc_dq]
  [ig_abc] -> "Frequency Droop (iabc -> id)"/1(iabc)
  [ig_dq] -> PQ Calculation (dq-Frame)/2(idq)
  PQ Calculation (dq-Frame)/1(pq) -> [pq]
  [vc_dq] -> PQ Calculation (dq-Frame)/1(vdq)
  "Frequency Droop (iabc -> id)"/1(w) -> [w]
  "Frequency Droop (iabc -> id)"/2(theta) -> [theta]
  [theta] -> "abc -> dq (Power-Invariant)2"/2(theta)
  [ig_abc] -> "abc -> dq (Power-Invariant)2"/1(abc)
  [il_abc] -> "abc -> dq (Power-Invariant)1"/1(abc)
  [vc_abc] -> "abc -> dq (Power-Invariant)"/1(abc)
  [theta] -> "abc -> dq (Power-Invariant)1"/2(theta)
  [theta] -> "abc -> dq (Power-Invariant)"/2(theta)
  Bus Creator3/1 -> m/1
  Demux1/1 -> "Frequency Droop (iabc -> id)"/2(p)
  [pq] -> Demux1/1
  Bus Selector1/3 -> Gain4/1  "<igabc>"
  Bus Selector1/2 -> Gain3/1  "<ilabc>"
  Bus Selector1/1 -> Gain2/1  "<vcabc>"
  Gain4/1 -> [ig_abc]  "w"
  [m_filter] -> Bus Selector1/1
  Gain2/1 -> [vc_abc]  "w"
  Gain3/1 -> [il_abc]  "w"
  P_dc/1 -> [Pref], Divide/1
  Vdc/1 -> Scope1/1, [Vdc]
  [iout] -> Unit Delay3/1
  Divide3/1 -> [iout]
  [iin] -> Unit Delay2/1
  LCL Filter1/1(m) -> [m_filter]
  Divide/1 -> [iin]
  Demux2/2 -> vb1/1
  Gain6/1 -> Unit Delay1/1
  Unit Delay3/1 -> Controlled Current Source/1
  Demux2/3 -> vc1/1
  Unit Delay1/1 -> Demux2/1
  Unit Delay2/1 -> Controlled Current Source1/1
  Demux2/1 -> va1/1
  [Vdc] -> Divide3/2
  [Vdc] -> Divide/2
  [Pref] -> "Frequency Droop (iabc -> id)"/3(Pref)
  Math Function/1 -> Sum3/2
  Constant3/1 -> Sum3/1
  [Vdc] -> Math Function/1
  Sum3/1 -> "Frequency Droop (iabc -> id)"/4(eDC)
  [Vdc] -> Bus Creator3/12  "Vdc"
  [vi_abc] -> Gain6/1
  Constant/1 -> Current Controller/4(enable)
  Current Controller/1(vidq*) -> [vi_dq], "dq -> abc (Power-Invariant)"/1(dq)
  [vc_dq] -> Voltage Controller/2(vcdq)
  [vc_dq] -> Current Controller/3(vdq)
  [il_dq] -> Demux3/1, Current Controller/2(iIdq)
  [ig_dq] -> Voltage Controller/3(igdq)
  Voltage Controller/1(ildq*) -> Demux/1, Current Controller/1(iIdq*)
  Constant1/1 -> Voltage Controller/4(enable)
  "dq -> abc (Power-Invariant)"/1(abc) -> [vi_abc]
  [theta] -> "dq -> abc (Power-Invariant)"/2(theta)
  Bus Selector1/4 -> Gain5/1  "<viiabc>"
  Gain5/1 -> [vii_abc]  "w"
  P Calculation (abc-Frame)/1(p) -> Divide3/1
  [vii_abc] -> P Calculation (abc-Frame)/1(vabc)
  [il_abc] -> P Calculation (abc-Frame)/2(iabc)
  Mux/1 -> Scope/1
  Mux1/1 -> Scope/2
  Demux/1 -> Mux/1
  Demux3/1 -> Mux/2
  Demux/2 -> Mux1/1
  Demux3/2 -> Mux1/2
  Demux4/1 -> Gain7/1
  [ig_dq] -> Demux4/1
  vcdq*/1 -> Demux5/1
  Demux4/2 -> Gain8/1
  Gain8/1 -> Sum1/1
  Gain7/1 -> Sum/1
  Demux5/1 -> Sum/2
  Sum/1 -> Mux2/1
  Demux5/2 -> Sum1/2
  Sum1/1 -> Mux2/2
  Mux2/1 -> Voltage Controller/1(vcdq*)
  connections:
  Series RLC Branch/LConn1 -- Diode/LConn1 -- Controlled Current Source1/RConn1 -- Vdc/LConn1 -- Controlled Current Source/LConn1
  va1/LConn1 -- LCL Filter1/LConn4 -- N/RConn1 -- vc1/LConn1 -- vb1/LConn1
  Series RLC Branch/RConn1 -- Controlled Current Source1/LConn1 -- DC Voltage Source/LConn1 -- Controlled Current Source/RConn1 -- Vdc/LConn2
  LCL Filter1/LConn2 -- vb1/RConn1
  LCL Filter1/RConn1 -- a/RConn1
  LCL Filter1/LConn3 -- vc1/RConn1
  LCL Filter1/LConn1 -- va1/RConn1
  LCL Filter1/RConn2 -- b/RConn1
  LCL Filter1/RConn3 -- c/RConn1
  DC Voltage Source/RConn1 -- Diode/RConn1

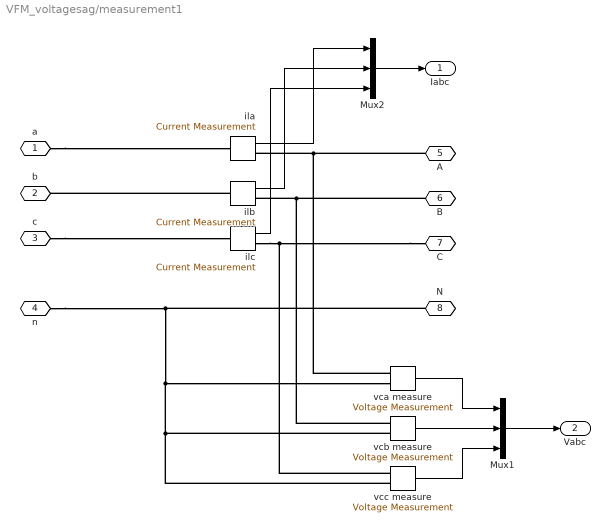
== system VFM_voltagesag/measurement1 ==
  Mux1 : Mux  Inputs=3
  Mux2 : Mux  Inputs=3
  ila : spsCurrentMeasurementLib/Current Measurement  PhasorSimulation=off  OutputType=Complex  PSBequivalent=0
  ilb : spsCurrentMeasurementLib/Current Measurement  PhasorSimulation=off  OutputType=Complex  PSBequivalent=0
  ilc : spsCurrentMeasurementLib/Current Measurement  PhasorSimulation=off  OutputType=Complex  PSBequivalent=0
  vca measure : spsVoltageMeasurementLib/Voltage Measurement  PhasorSimulation=off  OutputType=Complex  PSBequivalent=0
  vcb measure : spsVoltageMeasurementLib/Voltage Measurement  PhasorSimulation=off  OutputType=Complex  PSBequivalent=0
  vcc measure : spsVoltageMeasurementLib/Voltage Measurement  PhasorSimulation=off  OutputType=Complex  PSBequivalent=0
  a : PMIOPort  Side=Left
  b : PMIOPort  Port=2  Side=Left
  c : PMIOPort  Port=3  Side=Left
  n : PMIOPort  Port=4  Side=Left
  A : PMIOPort  Port=5  Side=Right
  B : PMIOPort  Port=6  Side=Right
  C : PMIOPort  Port=7  Side=Right
  N : PMIOPort  Port=8  Side=Right
  Iabc : Outport
  Vabc : Outport  Port=2
  wires:
  ila/1 -> Mux2/1
  ilb/1 -> Mux2/2
  ilc/1 -> Mux2/3
  Mux2/1 -> Iabc/1
  vcb measure/1 -> Mux1/2
  vca measure/1 -> Mux1/1
  vcc measure/1 -> Mux1/3
  Mux1/1 -> Vabc/1
  connections:
  a/RConn1 -- ila/LConn1
  ila/RConn1 -- A/RConn1 -- vca measure/LConn1
  ilb/LConn1 -- b/RConn1
  ilb/RConn1 -- B/RConn1 -- vcb measure/LConn1
  c/RConn1 -- ilc/LConn1
  C/RConn1 -- ilc/RConn1 -- vcc measure/LConn1
  n/RConn1 -- vcc measure/LConn2 -- vcb measure/LConn2 -- vca measure/LConn2 -- N/RConn1

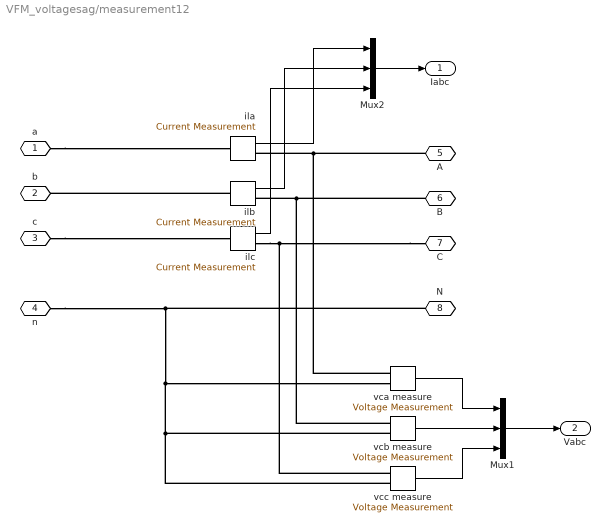
== system VFM_voltagesag/measurement12 ==
  Mux1 : Mux  Inputs=3
  Mux2 : Mux  Inputs=3
  ila : spsCurrentMeasurementLib/Current Measurement  PhasorSimulation=off  OutputType=Complex  PSBequivalent=0
  ilb : spsCurrentMeasurementLib/Current Measurement  PhasorSimulation=off  OutputType=Complex  PSBequivalent=0
  ilc : spsCurrentMeasurementLib/Current Measurement  PhasorSimulation=off  OutputType=Complex  PSBequivalent=0
  vca measure : spsVoltageMeasurementLib/Voltage Measurement  PhasorSimulation=off  OutputType=Complex  PSBequivalent=0
  vcb measure : spsVoltageMeasurementLib/Voltage Measurement  PhasorSimulation=off  OutputType=Complex  PSBequivalent=0
  vcc measure : spsVoltageMeasurementLib/Voltage Measurement  PhasorSimulation=off  OutputType=Complex  PSBequivalent=0
  a : PMIOPort  Side=Left
  b : PMIOPort  Port=2  Side=Left
  c : PMIOPort  Port=3  Side=Left
  n : PMIOPort  Port=4  Side=Left
  A : PMIOPort  Port=5  Side=Right
  B : PMIOPort  Port=6  Side=Right
  C : PMIOPort  Port=7  Side=Right
  N : PMIOPort  Port=8  Side=Right
  Iabc : Outport
  Vabc : Outport  Port=2
  wires:
  ila/1 -> Mux2/1
  ilb/1 -> Mux2/2
  ilc/1 -> Mux2/3
  Mux2/1 -> Iabc/1
  vcb measure/1 -> Mux1/2
  vca measure/1 -> Mux1/1
  vcc measure/1 -> Mux1/3
  Mux1/1 -> Vabc/1
  connections:
  a/RConn1 -- ila/LConn1
  ila/RConn1 -- A/RConn1 -- vca measure/LConn1
  ilb/LConn1 -- b/RConn1
  ilb/RConn1 -- B/RConn1 -- vcb measure/LConn1
  c/RConn1 -- ilc/LConn1
  C/RConn1 -- ilc/RConn1 -- vcc measure/LConn1
  n/RConn1 -- vcc measure/LConn2 -- vcb measure/LConn2 -- vca measure/LConn2 -- N/RConn1

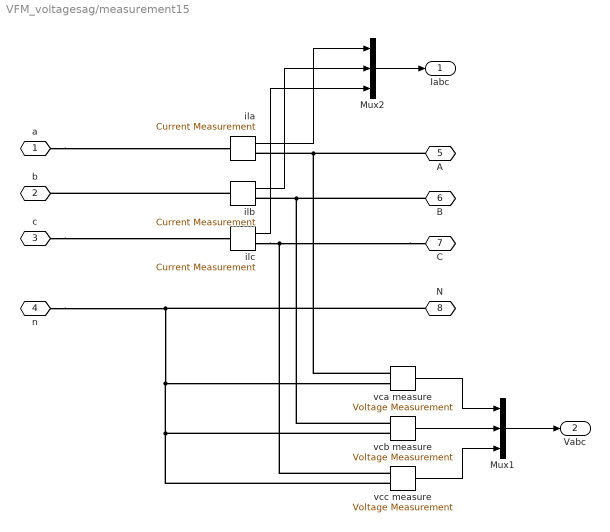
== system VFM_voltagesag/measurement15 ==
  Mux1 : Mux  Inputs=3
  Mux2 : Mux  Inputs=3
  ila : spsCurrentMeasurementLib/Current Measurement  PhasorSimulation=off  OutputType=Complex  PSBequivalent=0
  ilb : spsCurrentMeasurementLib/Current Measurement  PhasorSimulation=off  OutputType=Complex  PSBequivalent=0
  ilc : spsCurrentMeasurementLib/Current Measurement  PhasorSimulation=off  OutputType=Complex  PSBequivalent=0
  vca measure : spsVoltageMeasurementLib/Voltage Measurement  PhasorSimulation=off  OutputType=Complex  PSBequivalent=0
  vcb measure : spsVoltageMeasurementLib/Voltage Measurement  PhasorSimulation=off  OutputType=Complex  PSBequivalent=0
  vcc measure : spsVoltageMeasurementLib/Voltage Measurement  PhasorSimulation=off  OutputType=Complex  PSBequivalent=0
  a : PMIOPort  Side=Left
  b : PMIOPort  Port=2  Side=Left
  c : PMIOPort  Port=3  Side=Left
  n : PMIOPort  Port=4  Side=Left
  A : PMIOPort  Port=5  Side=Right
  B : PMIOPort  Port=6  Side=Right
  C : PMIOPort  Port=7  Side=Right
  N : PMIOPort  Port=8  Side=Right
  Iabc : Outport
  Vabc : Outport  Port=2
  wires:
  ila/1 -> Mux2/1
  ilb/1 -> Mux2/2
  ilc/1 -> Mux2/3
  Mux2/1 -> Iabc/1
  vcb measure/1 -> Mux1/2
  vca measure/1 -> Mux1/1
  vcc measure/1 -> Mux1/3
  Mux1/1 -> Vabc/1
  connections:
  a/RConn1 -- ila/LConn1
  ila/RConn1 -- A/RConn1 -- vca measure/LConn1
  ilb/LConn1 -- b/RConn1
  ilb/RConn1 -- B/RConn1 -- vcb measure/LConn1
  c/RConn1 -- ilc/LConn1
  C/RConn1 -- ilc/RConn1 -- vcc measure/LConn1
  n/RConn1 -- vcc measure/LConn2 -- vcb measure/LConn2 -- vca measure/LConn2 -- N/RConn1

== system VFM_voltagesag/measurement5 ==
  Mux1 : Mux  Inputs=3
  Mux2 : Mux  Inputs=3
  ila : spsCurrentMeasurementLib/Current Measurement  PhasorSimulation=off  OutputType=Complex  PSBequivalent=0
  ilb : spsCurrentMeasurementLib/Current Measurement  PhasorSimulation=off  OutputType=Complex  PSBequivalent=0
  ilc : spsCurrentMeasurementLib/Current Measurement  PhasorSimulation=off  OutputType=Complex  PSBequivalent=0
  vca measure : spsVoltageMeasurementLib/Voltage Measurement  PhasorSimulation=off  OutputType=Complex  PSBequivalent=0
  vcb measure : spsVoltageMeasurementLib/Voltage Measurement  PhasorSimulation=off  OutputType=Complex  PSBequivalent=0
  vcc measure : spsVoltageMeasurementLib/Voltage Measurement  PhasorSimulation=off  OutputType=Complex  PSBequivalent=0
  a : PMIOPort  Side=Left
  b : PMIOPort  Port=2  Side=Left
  c : PMIOPort  Port=3  Side=Left
  n : PMIOPort  Port=4  Side=Left
  A : PMIOPort  Port=5  Side=Right
  B : PMIOPort  Port=6  Side=Right
  C : PMIOPort  Port=7  Side=Right
  N : PMIOPort  Port=8  Side=Right
  Iabc : Outport
  Vabc : Outport  Port=2
  wires:
  ila/1 -> Mux2/1
  ilb/1 -> Mux2/2
  ilc/1 -> Mux2/3
  Mux2/1 -> Iabc/1
  vcb measure/1 -> Mux1/2
  vca measure/1 -> Mux1/1
  vcc measure/1 -> Mux1/3
  Mux1/1 -> Vabc/1
  connections:
  a/RConn1 -- ila/LConn1
  ila/RConn1 -- A/RConn1 -- vca measure/LConn1
  ilb/LConn1 -- b/RConn1
  ilb/RConn1 -- B/RConn1 -- vcb measure/LConn1
  c/RConn1 -- ilc/LConn1
  C/RConn1 -- ilc/RConn1 -- vcc measure/LConn1
  n/RConn1 -- vcc measure/LConn2 -- vcb measure/LConn2 -- vca measure/LConn2 -- N/RConn1
